simulink model "testsim_2016a"  (R2016a)
settings: Solver=ode4  StartTime=0.0  StopTime=4  FixedStep=0.001  RelTol=1e-3
libraries: simulink x5
settings Model: ExtModeTrigMode=oneshot  ExtModeArmWhenConnect=off  Creator=hp  LastModifiedBy=Administrator
settings SolverCC: AlgebraicLoopSolver=LineSearch
settings DataIOCC: SaveFormat=Array  SignalLoggingSaveFormat=ModelDataLogs  SignalLoggingName=sigsOut
settings OptimizationCC: BooleanDataType=off  ExpressionDepthLimit=2147483647  InitFltsAndDblsToZero=on
settings DebuggingCC: SaveWithParameterizedLinksMsg=none  UnderspecifiedInitializationDetection=Classic  MergeDetectMultiDrivingBlocksExec=none  SignalResolutionControl=TryResolveAllWithWarning  MultiTaskDSMMsg=warning  MultiTaskCondExecSysMsg=none  FcnCallInpInsideContextMsg=EnableAllAsWarning  StateNameClashWarn=warning
settings HardwareCC: ProdBitPerPointer=32  ProdLargestAtomicFloat=None  ProdIntDivRoundTo=Undefined  ProdEndianess=Unspecified  ProdWordSize=32  ProdHWDeviceType=32-bit Generic  TargetUnknown=on
settings ModelReferenceCC: PropagateSignalLabelsOutOfModel=off
settings GRTTargetCC: TargetFcnLib=ansi_tfl_tmw.mat  CombineOutputUpdateFcns=off  GRTInterface=on

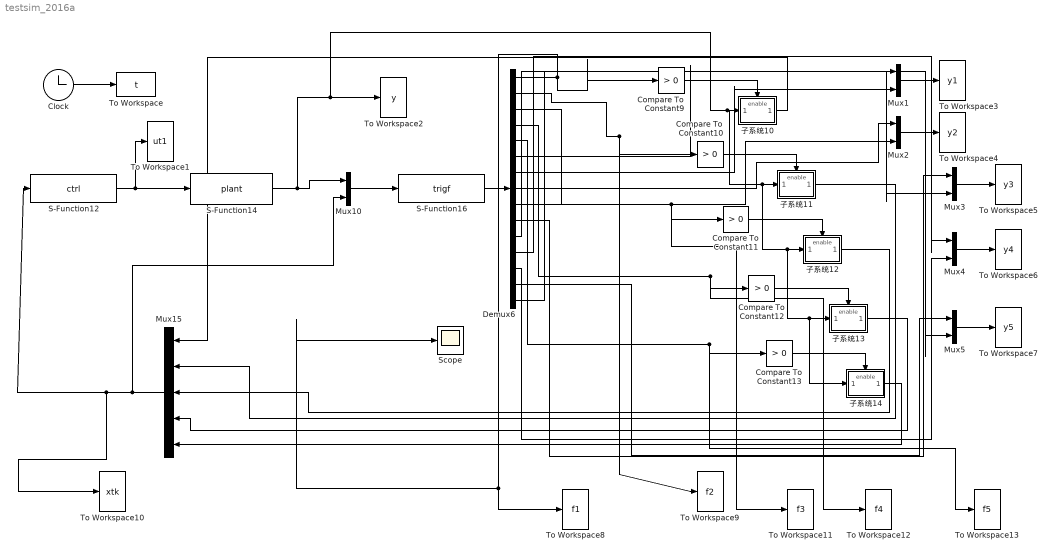
== system testsim_2016a ==
  Clock : Clock
  Compare To Constant{9..13} (5 alike) : simulink/Logic and Bit Operations/Compare To Constant  relop=>  const=0  OutDataTypeStr=boolean
  Demux6 : Demux  Outputs=15
  Mux{1..5,10} (6 alike) : Mux  Inputs=2
  Mux15 : Mux  Inputs=5
  S-Function12 : S-Function  FunctionName=ctrl  SFunctionDeploymentMode=off  EnableBusSupport=off
  S-Function14 : S-Function  FunctionName=plant  SFunctionDeploymentMode=off  EnableBusSupport=off
  S-Function16 : S-Function  FunctionName=trigf  SFunctionDeploymentMode=off  EnableBusSupport=off
  Scope : Scope
  To Workspace : ToWorkspace  VariableName=t  SampleTime=-1
  To Workspace1 : ToWorkspace  VariableName=ut1  SampleTime=-1
  To Workspace10 : ToWorkspace  VariableName=xtk  SampleTime=-1
  To Workspace11 : ToWorkspace  VariableName=f3  SampleTime=-1
  To Workspace12 : ToWorkspace  VariableName=f4  SampleTime=-1
  To Workspace13 : ToWorkspace  VariableName=f5  SampleTime=-1
  To Workspace2 : ToWorkspace  VariableName=y  SampleTime=-1
  To Workspace3 : ToWorkspace  VariableName=y1  SampleTime=-1
  To Workspace4 : ToWorkspace  VariableName=y2  SampleTime=-1
  To Workspace5 : ToWorkspace  VariableName=y3  SampleTime=-1
  To Workspace6 : ToWorkspace  VariableName=y4  SampleTime=-1
  To Workspace7 : ToWorkspace  VariableName=y5  SampleTime=-1
  To Workspace8 : ToWorkspace  VariableName=f1  SampleTime=-1
  To Workspace9 : ToWorkspace  VariableName=f2  SampleTime=-1
  子系统10 : Subsystem  TreatAsAtomicUnit=on
  子系统11 : Subsystem  TreatAsAtomicUnit=on
  子系统12 : Subsystem  TreatAsAtomicUnit=on
  子系统13 : Subsystem  TreatAsAtomicUnit=on
  子系统14 : Subsystem  TreatAsAtomicUnit=on
  wires:
  Clock/1 -> To Workspace/1
  S-Function12/1 -> To Workspace1/1, S-Function14/1
  Compare To Constant9/1 -> 子系统10/Enable
  Compare To Constant10/1 -> 子系统11/Enable
  Compare To Constant11/1 -> 子系统12/Enable
  Compare To Constant12/1 -> 子系统13/Enable
  Compare To Constant13/1 -> 子系统14/Enable
  子系统10/1(Out1) -> Mux15/1
  子系统12/1(Out1) -> Mux15/3
  子系统13/1(Out1) -> Mux15/4
  子系统14/1(Out1) -> Mux15/5
  Mux15/1 -> Mux10/2, To Workspace10/1, S-Function12/1
  子系统11/1(Out1) -> Mux15/2
  S-Function16/1 -> Demux6/1
  Mux10/1 -> S-Function16/1
  Mux1/1 -> To Workspace3/1
  Mux2/1 -> To Workspace4/1
  Mux3/1 -> To Workspace5/1
  Mux4/1 -> To Workspace6/1
  Mux5/1 -> To Workspace7/1
  Demux6/1 -> Compare To Constant9/1, To Workspace8/1, Scope/1
  Demux6/2 -> To Workspace9/1, Compare To Constant10/1
  Demux6/3 -> To Workspace11/1, Compare To Constant11/1
  Demux6/4 -> To Workspace12/1, Compare To Constant12/1
  Demux6/5 -> To Workspace13/1, Compare To Constant13/1
  Demux6/6 -> Mux1/1
  Demux6/7 -> Mux1/2
  Demux6/8 -> Mux2/1
  Demux6/9 -> Mux2/2
  Demux6/10 -> Mux3/1
  Demux6/11 -> Mux3/2
  Demux6/12 -> Mux4/1
  Demux6/13 -> Mux4/2
  Demux6/14 -> Mux5/1
  Demux6/15 -> Mux5/2
  S-Function14/1 -> 子系统14/1(In1), 子系统13/1(In1), 子系统12/1(In1), 子系统11/1(In1), 子系统10/1(In1), To Workspace2/1, Mux10/1

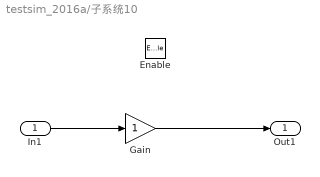
== system testsim_2016a/子系统10 ==
  In1 : Inport
  Enable : EnablePort
  Gain : Gain
  Out1 : Outport
  wires:
  In1/1 -> Gain/1
  Gain/1 -> Out1/1

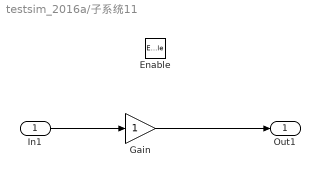
== system testsim_2016a/子系统11 ==
  In1 : Inport
  Enable : EnablePort
  Gain : Gain
  Out1 : Outport
  wires:
  Gain/1 -> Out1/1
  In1/1 -> Gain/1

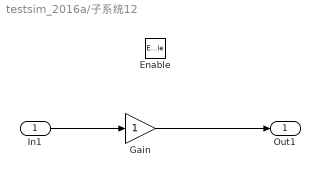
== system testsim_2016a/子系统12 ==
  In1 : Inport
  Enable : EnablePort
  Gain : Gain
  Out1 : Outport
  wires:
  In1/1 -> Gain/1
  Gain/1 -> Out1/1

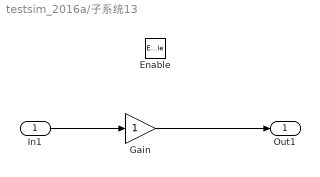
== system testsim_2016a/子系统13 ==
  In1 : Inport
  Enable : EnablePort
  Gain : Gain
  Out1 : Outport
  wires:
  Gain/1 -> Out1/1
  In1/1 -> Gain/1

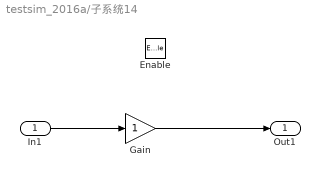
== system testsim_2016a/子系统14 ==
  In1 : Inport
  Enable : EnablePort
  Gain : Gain
  Out1 : Outport
  wires:
  In1/1 -> Gain/1
  Gain/1 -> Out1/1
